simulink model "simulink_ma"  (R2018a)
settings: Solver=ode45  StartTime=0.0  StopTime=1366  RelTol=1e-3
values from neighbouring files (symbols this model uses):
  ae = 329.2  / fator    (= 5.48666666667)    [carregaDadosDoModelo.m]    (also in carregaDadosSimulacao.m = 5.4867)
  anp = 16.5    [carregaDadosSimulacao.m]
  av = 414.17 / fator    (= 6.90283333333)    [carregaDadosDoModelo.m]    (also in carregaDadosSimulacao.m = 6.9028)
  K = 0.36783    [carregaDados.m]    (also in carregaDadosDoModelo.m = 0.01332; carregaDadosSimulacao.m = 0.01)
  Kc = 1       * fator    (= 60)    [carregaDadosDoModelo.m]    (also in carregaDadosSimulacao.m = 2.5)
  Ke = 0.395   * fator    (= 23.7)    [carregaDadosDoModelo.m]    (also in carregaDadosSimulacao.m = 1.4)
  Knp = 0.1    [carregaDadosSimulacao.m]
  Kr = 0.016835* fator    (= 1.0101)    [carregaDadosDoModelo.m]
  Ktp = 36.5    [carregaDadosSimulacao.m]
  Kv = 0.647   * fator    (= 38.82)    [carregaDadosDoModelo.m]    (also in carregaDadosSimulacao.m = 3.3)
  td = 0.065    [carregaDados.m]    (also in carregaDadosSimulacao.m = 5)
settings Model: Creator=root  LastModifiedBy=alexa
settings DataIOCC: LimitDataPoints=on  SaveFormat=Array
settings OptimizationCC: BlockReduction=off  BooleanDataType=off  LifeSpan=inf
settings DebuggingCC: SaveWithParameterizedLinksMsg=none  UnderspecifiedInitializationDetection=Classic  MergeDetectMultiDrivingBlocksExec=none  SignalResolutionControl=TryResolveAllWithWarning  SFUnexpectedBacktrackingDiag=warning  SFNoUnconditionalDefaultTransitionDiag=warning  SFExecutionAtInitializationDiag=none
settings HardwareCC: ProdBitPerPointer=32  ProdBitPerSizeT=32  ProdBitPerPtrDiffT=32  ProdLargestAtomicFloat=None  ProdIntDivRoundTo=Undefined  ProdEndianess=Unspecified  ProdWordSize=32  ProdHWDeviceType=32-bit Generic  TargetUnknown=on
settings ModelReferenceCC: PropagateSignalLabelsOutOfModel=off
settings CodeAppCC: StateflowObjectComments=on
settings GRTTargetCC: TargetLangStandard=C89/C90 (ANSI)  GeneratePreprocessorConditionals=Disable all
settings ConfigComp: CovMetricSettings=dw  CovHtmlReporting=on  CovSaveCumulativeToWorkspaceVar=on  CovSaveSingleToWorkspaceVar=on  CovExternalEMLEnable=off

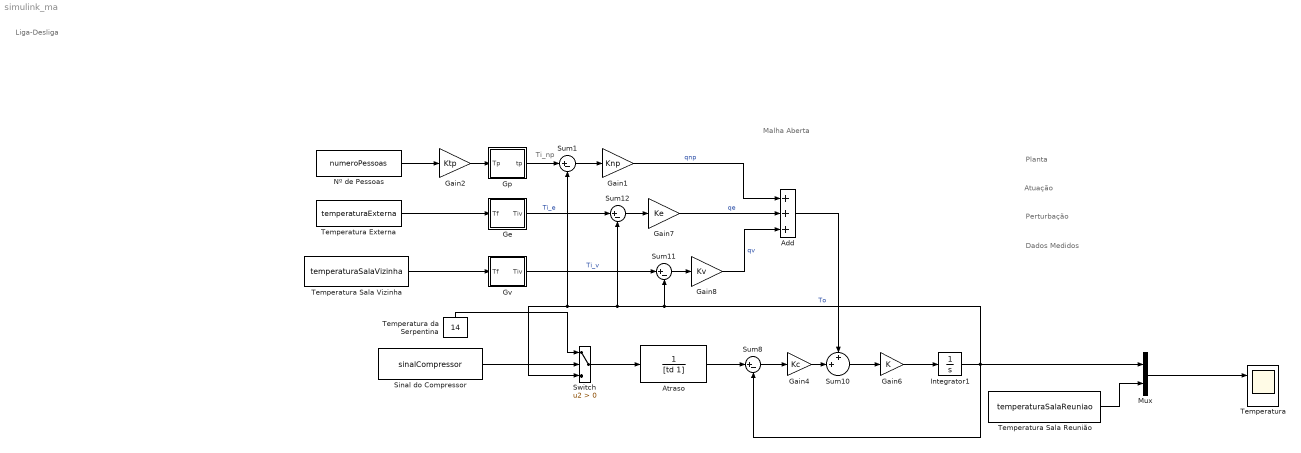
== system simulink_ma ==
  note: Planta
  note: Ti_np
  note: Perturbação
  note: Atuação
  note: Dados Medidos
  note: Liga-Desliga
  note: Malha Aberta
  Add : Sum  Inputs=+++
  Atraso : TransferFcn  Denominator=[td 1]
  Gain1 : Gain  Gain=Knp
  Gain2 : Gain  Gain=Ktp
  Gain4 : Gain  Gain=Kc
  Gain6 : Gain  Gain=K
  Gain7 : Gain  Gain=Ke
  Gain8 : Gain  Gain=Kv
  Ge : Subsystem
  Gp : Subsystem
  Gv : Subsystem
  Integrator1 : Integrator  InitialCondition=24
  Mux : Mux  Inputs=2
  Nº de Pessoas : FromWorkspace  VariableName=numeroPessoas  SampleTime=1
  Sinal do Compressor : FromWorkspace  VariableName=sinalCompressor  SampleTime=1
  Sum{1,8,11..12} (4 alike) : Sum  Inputs=|+-
  Sum10 : Sum  Inputs=++|
  Switch : Switch  Criteria=u2 > Threshold
  Temperatura : Scope  NumInputPorts=2
  Temperatura da Serpentina : Constant  Value=14
  Temperatura Externa : FromWorkspace  VariableName=temperaturaExterna  SampleTime=1
  "Temperatura Sala Reunião " : FromWorkspace  VariableName=temperaturaSalaReuniao  SampleTime=1
  Temperatura Sala Vizinha : FromWorkspace  VariableName=temperaturaSalaVizinha  SampleTime=1
  wires:
  Gain6/1 -> Integrator1/1
  Sum8/1 -> Gain4/1
  Gain4/1 -> Sum10/2
  Sum10/1 -> Gain6/1
  Sum12/1 -> Gain7/1
  Ge/1(Tiv) -> Sum12/1  "Ti_e"
  Integrator1/1 -> Mux/1, Switch/3, Sum1/2, Sum12/2, Sum11/2, Sum8/2  "To"
  Sum11/1 -> Gain8/1
  Gv/1(Tiv) -> Sum11/1  "Ti_v"
  Temperatura Sala Vizinha/1 -> Gv/1(Tf)
  Add/1 -> Sum10/1
  Temperatura da Serpentina/1 -> Switch/1
  Atraso/1 -> Sum8/1
  Temperatura Externa/1 -> Ge/1(Tf)
  Switch/1 -> Atraso/1
  Sinal do Compressor/1 -> Switch/2
  Mux/1 -> Temperatura/1
  Gp/1("tp ") -> Sum1/1
  Sum1/1 -> Gain1/1
  Nº de Pessoas/1 -> Gain2/1
  Gain2/1 -> Gp/1(Tp)
  Gain8/1 -> Add/3  "qv"
  Gain7/1 -> Add/2  "qe"
  "Temperatura Sala Reunião "/1 -> Mux/2
  Gain1/1 -> Add/1  "qnp"

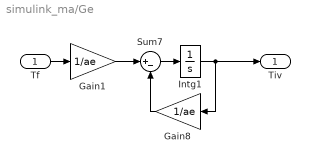
== system simulink_ma/Ge ==
  Tf : Inport
  Gain1 : Gain  Gain=1/ae
  Gain8 : Gain  Gain=1/ae
  Intg1 : Integrator  InitialCondition=30
  Sum7 : Sum  Inputs=|+-
  Tiv : Outport
  wires:
  Gain1/1 -> Sum7/1
  Tf/1 -> Gain1/1
  Gain8/1 -> Sum7/2
  Intg1/1 -> Tiv/1, Gain8/1
  Sum7/1 -> Intg1/1

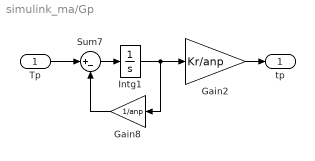
== system simulink_ma/Gp ==
  Tp : Inport
  Gain2 : Gain  Gain=Kr/anp
  Gain8 : Gain  Gain=1/anp
  Intg1 : Integrator
  Sum7 : Sum  Inputs=|+-
  "tp " : Outport
  wires:
  Gain2/1 -> "tp "/1
  Tp/1 -> Sum7/1
  Gain8/1 -> Sum7/2
  Intg1/1 -> Gain2/1, Gain8/1
  Sum7/1 -> Intg1/1

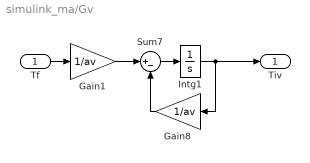
== system simulink_ma/Gv ==
  Tf : Inport
  Gain1 : Gain  Gain=1/av
  Gain8 : Gain  Gain=1/av
  Intg1 : Integrator  InitialCondition=30
  Sum7 : Sum  Inputs=|+-
  Tiv : Outport
  wires:
  Gain1/1 -> Sum7/1
  Tf/1 -> Gain1/1
  Gain8/1 -> Sum7/2
  Intg1/1 -> Tiv/1, Gain8/1
  Sum7/1 -> Intg1/1
